simulink model "balancingControllerWithHandControl"
settings: Solver=FixedStepDiscrete  StartTime=0.0  StopTime=inf  FixedStep=Ts  RelTol=1e-3
InitFcn:
  | initBalancingControllerWithHandControl;
values from neighbouring files (symbols this model uses):
  Rf = [R, zeros(3,3); zeros(3,3), R]    [initBalancingController.m]    (also in initBalancingControllerWithNonLinearImpedances.m; initBalancingController_QP.m)
undefined symbols (not defined in the file or in its folder): DiscIntNeverNeededParam, DT, kCom, kImp, kw, qFin
libraries: WBCLibrary x23, simulink x2, dspsigops x2
settings Model: Creator=daniele  LastModifiedBy=morteza
settings DataIOCC: LimitDataPoints=on  SaveFormat=Array  ReturnWorkspaceOutputs=off
settings OptimizationCC: ExpressionDepthLimit=2147483647  LifeSpan=inf  SimCompilerOptimization=Off
settings DebuggingCC: UnderspecifiedInitializationDetection=Classic  MergeDetectMultiDrivingBlocksExec=none  SolverPrmCheckMsg=warning  MultiTaskDSMMsg=warning  MultiTaskCondExecSysMsg=none  FcnCallInpInsideContextMsg=Enable All  FrameProcessingCompatibilityMsg=warning  StateNameClashWarn=warning  StrictBusMsg=None  SFUnexpectedBacktrackingDiag=warning  SFNoUnconditionalDefaultTransitionDiag=warning
settings HardwareCC: ProdBitPerPointer=32  ProdLargestAtomicFloat=None  ProdIntDivRoundTo=Undefined  ProdEndianess=Unspecified  ProdWordSize=32  ProdHWDeviceType=32-bit Generic
settings ModelReferenceCC: PropagateSignalLabelsOutOfModel=off
settings SFSimCC: SimUseLocalCustomCode=off
settings RTWCC: RTWUseLocalCustomCode=off  IncludeERTFirstTime=on  RTWCompilerOptimization=Off
settings CodeAppCC: CustomSymbolStrType=$N$R$M
settings GRTTargetCC: CodeReplacementLibrary=ANSI_C  GeneratePreprocessorConditionals=Disable all  CombineOutputUpdateFcns=off  CPPClassGenCompliant=off  GRTInterface=on

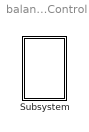
== system balancingControllerWithHandControl ==
  Subsystem : Subsystem  mask{robotName='iCubGenova01', Ts=0.01, localName='dynamicBalancing'}
      mask prompts: robotName "robot name"; localName "module name"

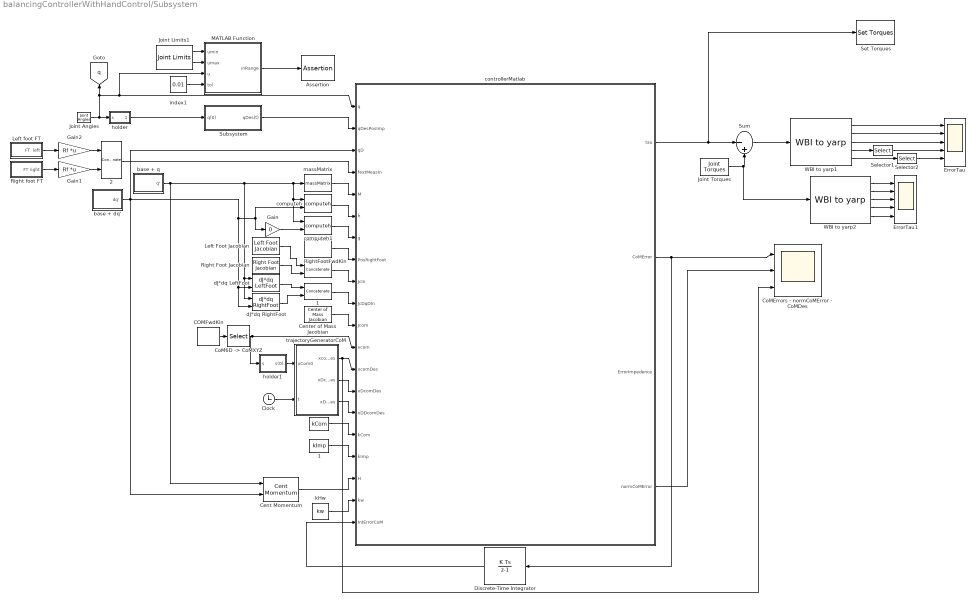
== system balancingControllerWithHandControl/Subsystem ==
  " " : Constant  Value=kCom
  " 1" : Constant  Value=kImp
  " " : Concatenate  Mode=Multidimensional array
  " 1" : Concatenate  Mode=Multidimensional array
  " 2" : Concatenate  Mode=Multidimensional array
  Assertion : Assertion  Enabled=on
  "COMFwdKin " : WBCLibrary/wholeBodyModel/Forward Kinematics/COMFwdKin   robotName=robotName  localName=localName
  Cent Momentum : WBCLibrary/wholeBodyModel/Dynamics/Cent Momentum  robotName=robotName  localName=localName
  Center of Mass Jacobian : WBCLibrary/wholeBodyModel/Jacobians/Center of Mass Jacobian  robotName=robotName  localName=localName
  Clock : Clock
  "CoM6D -> CoMXYZ" : Selector  InputPortWidth=7  IndexOptions=Index vector (dialog)  Indices=[1 2 3]  OutputSizes=1
  "CoMErrors - normCoMError - CoMDes " : Scope  NumInputPorts=3
      settings: TimeRange=1.6  YMin=-0.025~0~-5  YMax=0.005~0.04~5  SaveName=ScopeData6
  Discrete-Time Integrator : DiscreteIntegrator  InitialCondition=[0 0 0]  SampleTime=Ts  ICPrevOutput=DiscIntNeverNeededParam  ICPrevScaledInput=DiscIntNeverNeededParam
  ErrorTau : Scope  NumInputPorts=5
      settings: YMin=-12~-5~-5~-5~-5  YMax=12~5~5~5~5
  ErrorTau1 : Scope  NumInputPorts=5
      settings: YMin=-12~-5~-5~-5~-5  YMax=12~5~5~5~5
  Gain : Gain  Gain=0
  Gain1 : Gain  Gain=Rf  Multiplication=Matrix(K*u)
  Gain2 : Gain  Gain=Rf  Multiplication=Matrix(K*u)
  Joint Angles : WBCLibrary/wholeBodyStates/Joint Angles  robotName=robotName  localName=localName
  Joint Limits1 : WBCLibrary/wholeBodyModel/Joint Limits  robotName=robotName  localName=localName
  Joint Torques : WBCLibrary/wholeBodyStates/Joint Torques  robotName=robotName  localName=localName
  Left Foot Jacobian : WBCLibrary/wholeBodyModel/Jacobians/Left Foot Jacobian  robotName=robotName  localName=localName
  Left foot FT : Subsystem
  MATLAB Function : MATLAB Function  TreatAsAtomicUnit=on
  Right Foot Jacobian : WBCLibrary/wholeBodyModel/Jacobians/Right Foot Jacobian  robotName=robotName  localName=localName
  Right foot FT : Subsystem
  RightFootFwdKin : WBCLibrary/wholeBodyModel/Forward Kinematics/RightFootFwdKin  robotName=robotName  localName=localName
  Selector1 : Selector  InputPortWidth=6  IndexOptions=Index vector (dialog)  Indices=[2 5 ]  OutputSizes=1
  Selector2 : Selector  InputPortWidth=6  IndexOptions=Index vector (dialog)  Indices=[2 5 ]  OutputSizes=1
  Set Torques : WBCLibrary/wholeBodyActuators/Set Torques  val=6  robotName=robotName  localName=localName
  Subsystem : Subsystem
  Sum : Sum  Inputs=|-+
  WBI to yarp1 : WBCLibrary/Utilities/WBI to yarp
  WBI to yarp2 : WBCLibrary/Utilities/WBI to yarp
  base + dq' : Subsystem
  base + q : Subsystem
  computeh : WBCLibrary/wholeBodyModel/Dynamics/computeh  val=7  robotname=robotName  localname=localName
  computeh1 : WBCLibrary/wholeBodyModel/Dynamics/computeh  val=7  robotname=robotName  localname=localName
  controllerMatlab : MATLAB Function  TreatAsAtomicUnit=on
  dJ*dq LeftFoot : WBCLibrary/wholeBodyModel/Dynamics/dJ*dq LeftFoot  val=9  robotName=robotName  localName=localName
  dJ*dq RightFoot : WBCLibrary/wholeBodyModel/Dynamics/dJ*dq RightFoot  val=9  robotName=robotName  localName=localName
  holder : Subsystem
  holder1 : Subsystem
  index1 : Constant  Value=0.01  VectorParams1D=off
  kHw : Constant  Value=kw
  massMatrix : WBCLibrary/wholeBodyModel/Dynamics/massMatrix  val=8  robotname=robotName  localname=localName
  trajectoryGeneratorCoM : MATLAB Function  TreatAsAtomicUnit=on
  tag scope: q=global
  wires:
  computeh/1 -> controllerMatlab/6(h)
  massMatrix/1 -> controllerMatlab/5(M)
  Center of Mass Jacobian/1 -> controllerMatlab/11(Jcom)
  " "/1 -> controllerMatlab/16(kCom)
  Left Foot Jacobian/1 -> " "/1
  Right Foot Jacobian/1 -> " "/2
  trajectoryGeneratorCoM/1(xcomDes) -> "CoMErrors - normCoMError - CoMDes "/3, controllerMatlab/13(xcomDes)
  trajectoryGeneratorCoM/2(xDcomDes) -> controllerMatlab/14(xDcomDes)
  trajectoryGeneratorCoM/3(xDDcomDes) -> controllerMatlab/15(xDDcomDes)
  Clock/1 -> trajectoryGeneratorCoM/2(t)
  holder1/1(s(0)) -> trajectoryGeneratorCoM/1(xCom0)
  dJ*dq LeftFoot/1 -> " 1"/1
  dJ*dq RightFoot/1 -> " 1"/2
  "COMFwdKin "/1 -> "CoM6D -> CoMXYZ"/1
  "CoM6D -> CoMXYZ"/1 -> holder1/1(s), controllerMatlab/12(xcom)
  RightFootFwdKin/1 -> controllerMatlab/8(PosRightFoot)
  Discrete-Time Integrator/1 -> controllerMatlab/20(IntErrorCoM)
  base + q/1(q') -> dJ*dq RightFoot/1, dJ*dq LeftFoot/1, computeh1/1, computeh/1, massMatrix/1, Cent Momentum/1
  base + dq'/1(dq') -> dJ*dq RightFoot/2, dJ*dq LeftFoot/2, computeh/2, Gain/1, Cent Momentum/2, controllerMatlab/3(qD)
  Cent Momentum/1 -> controllerMatlab/18(H)
  kHw/1 -> controllerMatlab/19(kw)
  " 1"/1 -> controllerMatlab/10(JcDqDIn)
  " "/1 -> controllerMatlab/9(JcIn)
  Joint Torques/1 -> WBI to yarp2/1, Sum/2
  WBI to yarp1/1 -> ErrorTau/1
  WBI to yarp1/2 -> ErrorTau/2
  WBI to yarp1/3 -> ErrorTau/3
  WBI to yarp1/4 -> Selector1/1
  WBI to yarp1/5 -> Selector2/1
  controllerMatlab/1(tau) -> Set Torques/1, Sum/1
  Joint Limits1/1 -> MATLAB Function/1(umin)
  Joint Limits1/2 -> MATLAB Function/2(umax)
  Joint Angles/1 -> MATLAB Function/3(u), controllerMatlab/1(q), [q], holder/1(s)
  index1/1 -> MATLAB Function/4(tol)
  controllerMatlab/2(CoMError) -> Discrete-Time Integrator/1, "CoMErrors - normCoMError - CoMDes "/1
  controllerMatlab/4(normCoMError) -> "CoMErrors - normCoMError - CoMDes "/2
  computeh1/1 -> controllerMatlab/7(g)
  Gain/1 -> computeh1/2
  " 1"/1 -> controllerMatlab/17(kImp)
  Right foot FT/1(FT right) -> Gain1/1
  Left foot FT/1(FT  left) -> Gain2/1
  Gain2/1 -> " 2"/1
  Gain1/1 -> " 2"/2
  " 2"/1 -> controllerMatlab/4(fextMeasIn)
  Sum/1 -> WBI to yarp1/1
  Subsystem/1(qDes(t)) -> controllerMatlab/2(qDesPosImp)
  holder/1(s(0)) -> Subsystem/1(q(0))
  MATLAB Function/1(inRange) -> Assertion/1
  WBI to yarp2/1 -> ErrorTau1/1
  WBI to yarp2/2 -> ErrorTau1/2
  WBI to yarp2/3 -> ErrorTau1/3
  WBI to yarp2/4 -> ErrorTau1/4
  WBI to yarp2/5 -> ErrorTau1/5
  Selector1/1 -> ErrorTau/4
  Selector2/1 -> ErrorTau/5

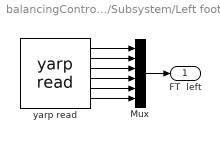
== system balancingControllerWithHandControl/Subsystem/Left foot FT ==
  Mux : Mux  Inputs=6
  yarp read : WBCLibrary/Utilities/yarp read  from='/wholeBodyDyanmicsTree/left_leg/endEffectorWrench:o'  to='...'  num=6
  FT  left : Outport
  wires:
  yarp read/1 -> Mux/1
  yarp read/2 -> Mux/2
  yarp read/3 -> Mux/3
  yarp read/4 -> Mux/4
  yarp read/5 -> Mux/5
  yarp read/6 -> Mux/6
  Mux/1 -> FT  left/1

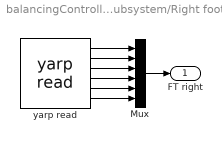
== system balancingControllerWithHandControl/Subsystem/Right foot FT ==
  Mux : Mux  Inputs=6
  yarp read : WBCLibrary/Utilities/yarp read  from='/wholeBodyDyanmicsTree/right_leg/endEffectorWrench:o'  to='...'  num=6
  FT right : Outport
  wires:
  yarp read/1 -> Mux/1
  yarp read/2 -> Mux/2
  yarp read/3 -> Mux/3
  yarp read/4 -> Mux/4
  yarp read/5 -> Mux/5
  yarp read/6 -> Mux/6
  Mux/1 -> FT right/1

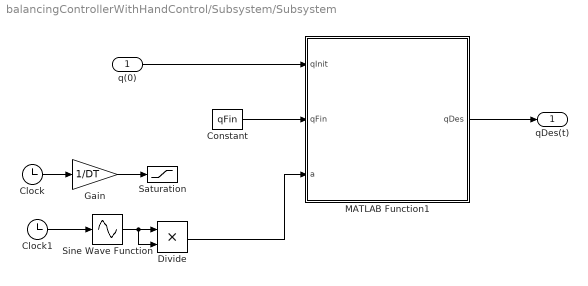
== system balancingControllerWithHandControl/Subsystem/Subsystem ==
  q(0) : Inport
  Clock : Clock
  Clock1 : Clock
  Constant : Constant  Value=qFin
  Divide : Product  Inputs=**
  Gain : Gain  Gain=1/DT
  MATLAB Function1 : MATLAB Function  TreatAsAtomicUnit=on
  Saturation : Saturate  UpperLimit=1  LowerLimit=0  SampleTime=Ts
  Sine Wave Function : Sin  TimeSource=Use external signal  Frequency=pi/DT  SampleTime=0
  qDes(t) : Outport
  wires:
  q(0)/1 -> MATLAB Function1/1(qInit)
  MATLAB Function1/1(qDes) -> qDes(t)/1
  Constant/1 -> MATLAB Function1/2(qFin)
  Clock/1 -> Gain/1
  Gain/1 -> Saturation/1
  Clock1/1 -> Sine Wave Function/1
  Sine Wave Function/1 -> Divide/2, Divide/1
  Divide/1 -> MATLAB Function1/3(a)

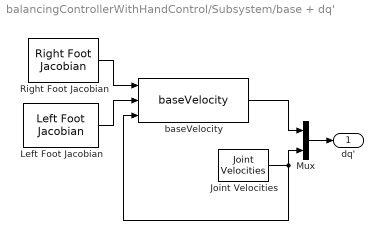
== system balancingControllerWithHandControl/Subsystem/base + dq' ==
  Joint Velocities : WBCLibrary/wholeBodyStates/Joint Velocities  robotName=robotName  localName=localName
  Left Foot Jacobian : WBCLibrary/wholeBodyModel/Jacobians/Left Foot Jacobian  robotName=robotName  localName=localName
  Mux : Mux  Inputs=2
  Right Foot Jacobian : WBCLibrary/wholeBodyModel/Jacobians/Right Foot Jacobian  robotName=robotName  localName=localName
  baseVelocity : WBCLibrary/Utilities/baseVelocity
  dq' : Outport
  wires:
  Left Foot Jacobian/1 -> baseVelocity/2
  Right Foot Jacobian/1 -> baseVelocity/1
  baseVelocity/1 -> Mux/1
  Joint Velocities/1 -> baseVelocity/3, Mux/2
  Mux/1 -> dq'/1

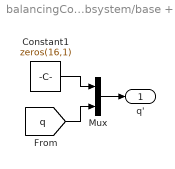
== system balancingControllerWithHandControl/Subsystem/base + q ==
  Constant1 : Constant  Value=zeros(16,1)
  Mux : Mux  Inputs=2
  q' : Outport
  wires:
  Mux/1 -> q'/1
  [q] -> Mux/2
  Constant1/1 -> Mux/1

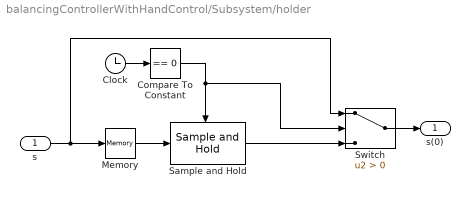
== system balancingControllerWithHandControl/Subsystem/holder ==
  s : Inport
  Clock : Clock
  Compare To Constant : simulink/Logic and Bit Operations/Compare To Constant  relop===  const=0  OutDataTypeStr=boolean
  Memory : Memory
  Sample and Hold : dspsigops/Sample and Hold  trig=Falling edge  initCond=0  latchinput=off
  Switch : Switch  Criteria=u2 > Threshold
  s(0) : Outport
  wires:
  s/1 -> Switch/1, Memory/1
  Clock/1 -> Compare To Constant/1
  Compare To Constant/1 -> Sample and Hold/Trigger, Switch/2
  Sample and Hold/1 -> Switch/3
  Switch/1 -> s(0)/1
  Memory/1 -> Sample and Hold/1

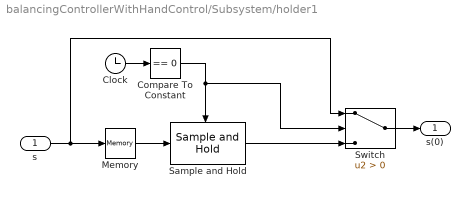
== system balancingControllerWithHandControl/Subsystem/holder1 ==
  s : Inport
  Clock : Clock
  Compare To Constant : simulink/Logic and Bit Operations/Compare To Constant  relop===  const=0  OutDataTypeStr=boolean
  Memory : Memory
  Sample and Hold : dspsigops/Sample and Hold  trig=Falling edge  initCond=0  latchinput=off
  Switch : Switch  Criteria=u2 > Threshold
  s(0) : Outport
  wires:
  s/1 -> Switch/1, Memory/1
  Clock/1 -> Compare To Constant/1
  Compare To Constant/1 -> Sample and Hold/Trigger, Switch/2
  Sample and Hold/1 -> Switch/3
  Switch/1 -> s(0)/1
  Memory/1 -> Sample and Hold/1

== matlab function balancingControllerWithHandControl/Subsystem/trajectoryGeneratorCoM ==
  data: xcomDes output; xDcomDes output; xDDcomDes output; xCom0 input; t input
function [xcomDes, xDcomDes, xDDcomDes] = fcn(xCom0,t)
%#codegen

e3 = [0;1;0];
A =  0.04;
f = 0.3;

xcomDes    = xCom0 + A*sin(2*pi*f*t)*e3;
xcomDes(3) =  xcomDes(3);
xDcomDes   =         A*2*pi*f*cos(2*pi*f*t)*e3;
xDDcomDes  =        -A*(2*pi*f)^2*sin(2*pi*f*t)*e3;

== matlab function balancingControllerWithHandControl/Subsystem/controllerMatlab ==
  data: q input; qDesPosImp input; qD input; fextMeasIn input; M input; h input; g input; PosRightFoot input; JcIn input; JcDqDIn input; tau output; Jcom input; xcom input; xcomDes input; xDcomDes input; xDDcomDes input; kCom input; kImp input; H input; kw input; CoMError output; IntErrorCoM input; ErrorImpedence output; normCoMError output
function [tau,CoMError,ErrorImpedence,normCoMError] = fcn(q,qDesPosImp,qD, fextMeasIn, M, h, g, PosRightFoot, JcIn, JcDqDIn, Jcom, xcom, xcomDes, xDcomDes, xDDcomDes, kCom, kImp ,H, kw,IntErrorCoM)
%#codegen

PINV_TOL = 1e-5;
gravAcc        = 9.81;

n = 25;
St    = [zeros(6,n);eye(n,n)];

m     = M(1,1);
grav = [zeros(2,1);-m*gravAcc;zeros(3,1)];

% Definition of reference accelerations for CoM and Joints that ensure
% stabilization of desired trajectories xDcomDes and qDes 

xDcom      = Jcom(1:3,:)*qD;
xDDcomStar = xDDcomDes - kCom(1)*(xcom - xcomDes) - kCom(2)*IntErrorCoM - kCom(3)*(xDcom - xDcomDes)  ;

Pr =  PosRightFoot(1:3) - xcom; % Application point of the contact force on the right foot w.r.t. CoM

A  = [ eye(3),   zeros(3),eye(3), zeros(3);
      -Sf(xcom),  eye(3), Sf(Pr), eye(3) ];
hwDotDes = H(4:end);
hDotDes  = [ m*xDDcomStar ;
             -kw*hwDotDes  ]; 
Jc = JcIn;         
JcDqD = JcDqDIn;
fextMeas = fextMeasIn;

% Jc    = [JcIn(1:3,:);JcIn(7:9,:)];       
% JcDqD = [JcDqDIn(1:3,:);JcDqDIn(7:9,:)];

% A  = [ eye(3),eye(3)];
% hDotDes  =  m*xDDcomStar; 
% fextMeas = [fextMeasIn(1:3);fextMeasIn(7:9)];

pinvA = pinv(A, PINV_TOL);
fd    = pinvA*(hDotDes-grav) ;% + (eye(length(fextMeas)) - pinvA*A)*fextMeas;

Minv = inv(M);
JcMinv        = Jc*Minv;
PInv_JcMinvSt = pinv(JcMinv*St, PINV_TOL);
N0            = eye(n) - PInv_JcMinvSt*JcMinv*St;

fextMeas = fd;

tau1 = PInv_JcMinvSt*(JcMinv*h - JcDqD - JcMinv*Jc'*fd);
LinearizedDynamics = g(7:end)-Jc(:,7:end)'*fextMeas - kImp.*(q-qDesPosImp);% - tau1 -diag(kDam)*N0'*qD(7:end) ;  %-kDam.*qD(7:end) 

tau0 = LinearizedDynamics;

tau = tau1 + N0*tau0;

% f = (JcMinv*Jc')^-1*(JcMinv*(h-[zeros(6,1);tau])-JcDqD);

CoMError    = xcom - xcomDes;
normCoMError  = norm(CoMError);
ErrorImpedence   = tau + LinearizedDynamics;

== matlab function balancingControllerWithHandControl/Subsystem/Subsystem/MATLAB Function1 ==
  data: qInit input; qFin input; qDes output; a input
function qDes = checkRange(qInit,qFin,a)
%#codegen
 
qFin(qFin == -5) = qInit(qFin == -5);

qDes = qInit + a*(qFin-qInit);

== matlab function balancingControllerWithHandControl/Subsystem/MATLAB Function ==
  data: umin input; umax input; u input; inRange output; tol input
function inRange = checkRange(umin, umax, u, tol)
%#codegen

res = u < umin + tol | u > umax - tol;
res = sum(res);
if res==0
    inRange = 1;
else
    inRange = 0;
    u < umin + tol | u > umax - tol
end
